simulink model "TangapCumTaoTai_2023b"  (R2023b)
settings: Solver=FixedStepAuto  StartTime=0  StopTime=350.02  FixedStep=0.00025  RelTol=1e-3  AbsTol=1e-3  EnableMultiTasking=on
undefined symbols (not defined in the file): Lg, rad, Rg, s
libraries: aerolibconvert2 x1, SignalEditorBlockLib x1
settings Model: Creator=Admin  LastModifiedBy=Legion
settings SolverCC: AutoScaleAbsTol=off  AlgebraicLoopSolver=TrustRegion  MaxZcPerStep=1
settings DataIOCC: LimitDataPoints=on  MaxDataPoints=10000
settings OptimizationCC: ReuseModelBlockBuffer=off  LifeSpan=inf
settings DebuggingCC: UnconnectedInputMsg=warning  UnconnectedOutputMsg=warning  UnconnectedLineMsg=warning  AllowSymbolicDim=off  SubsystemReferenceDiagnosticForUnitTest=warning  SFUnexpectedBacktrackingDiag=warning  SFNoUnconditionalDefaultTransitionDiag=warning  SFExecutionAtInitializationDiag=none  ArithmeticOperatorsInVariantConditions=warning
settings ModelReferenceCC: EnableRefExpFcnMdlSchedulingChecks=on
settings SFSimCC: SimUseLocalCustomCode=off  CustomCodeUndefinedFunction=UseInterfaceOnly
settings RTWCC: RTWUseLocalCustomCode=off  DLArmComputeVersion=19.05
settings CodeAppCC: StateflowObjectComments=on
settings GRTTargetCC: TargetLangStandard=C89/C90 (ANSI)
settings ConfigComp: CovMetricSettings=dw  CovSaveCumulativeToWorkspaceVar=on  CovSaveSingleToWorkspaceVar=on  CovExternalEMLEnable=off  CovSFcnEnable=off
settings SimscapeCC: SimscapeLogType=all  SimscapeLogSimulationStatistics=on  SimscapeLogDataHistory=10000

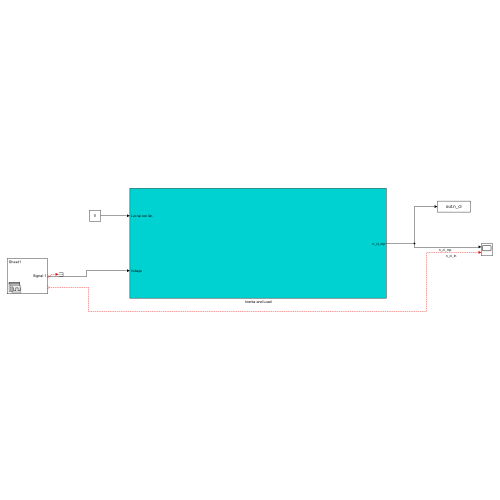
[thumbnail: Simulink's stored preview of the top-level diagram]
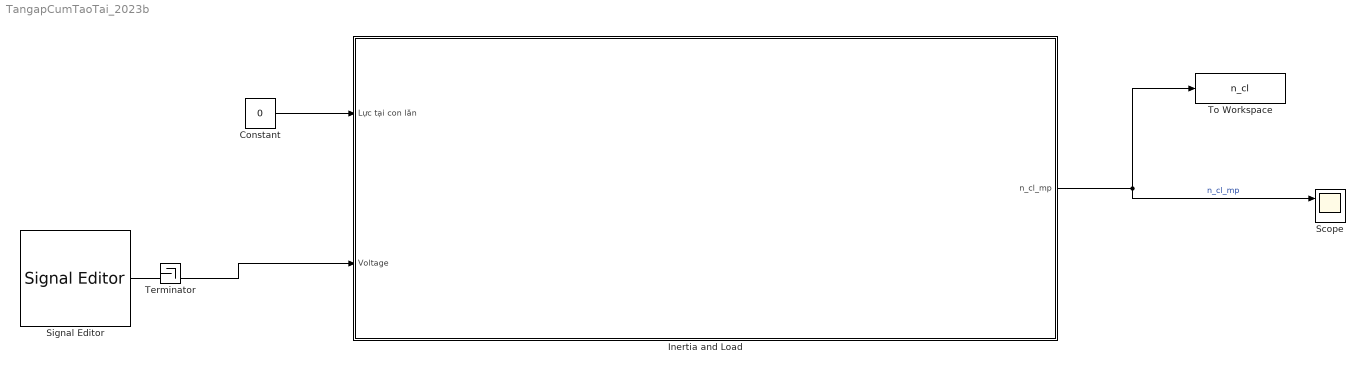
== system TangapCumTaoTai_2023b ==
  " Inertia and Load" : Subsystem
  Constant : Constant  Value=0
  Scope : Scope  NumInputPorts=2
  Signal Editor : SignalEditorBlockLib/Signal Editor  FileName=DataTangapcumtaotai.mat  ActiveScenario=Sheet1  ActiveSignal=Voltage  IsBus=off  OutputBusObjectStr=Bus: BusObject  SampleTime=0  ZeroCross=off  OutputAfterFinalValue=Setting to zero  Unit=inherit  PreserveSignalName=on  ApplySigPropsToAllScenarios=on  ApplySigPropsToAllSignals=off
  Terminator : Terminator
  To Workspace : ToWorkspace  VariableName=n_cl  SaveFormat=Timeseries  SampleTime=-1
  wires:
  Constant/1 -> " Inertia and Load"/1(Lực tại con lăn)
  Signal Editor/1 -> " Inertia and Load"/2(Voltage)
  ? -> Terminator/1
  " Inertia and Load"/1(n_cl_mp) -> To Workspace/1, Scope/1  "n_cl_mp"
  ? -> Scope/2  "n_cl_tn"

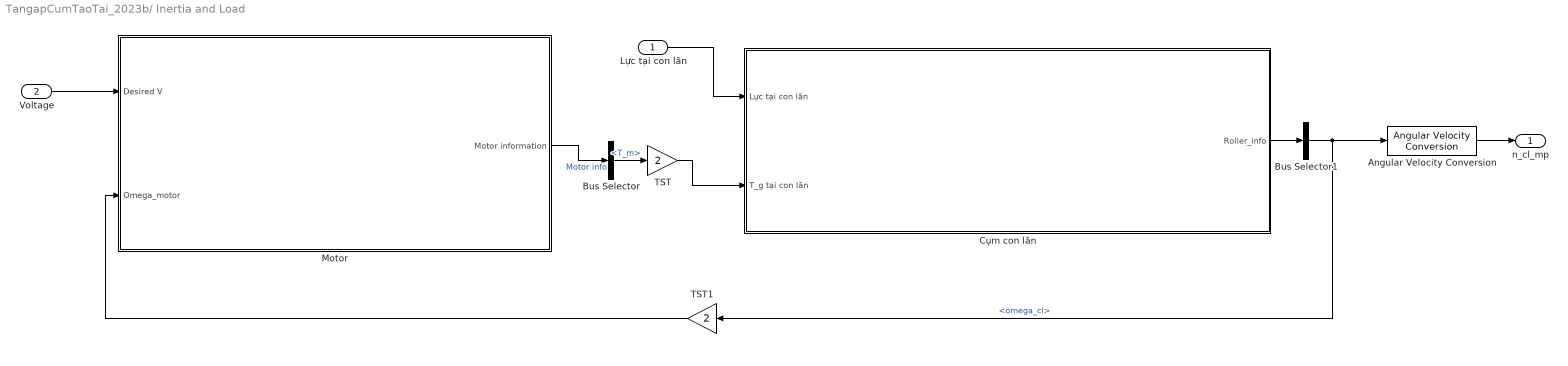
== system TangapCumTaoTai_2023b/ Inertia and Load ==
  Lực tại con lăn : Inport
  Voltage : Inport  Port=2
  Angular Velocity Conversion : aerolibconvert2/Angular Velocity Conversion  IU=rad/s  OU=rpm
  Bus Selector : BusSelector  OutputSignals=T_m
  Bus Selector1 : BusSelector  OutputSignals=omega_cl
  Cụm con lăn : Subsystem
  Motor : Subsystem
  TST : Gain  Gain=2
  TST1 : Gain  Gain=2
  n_cl_mp : Outport
  wires:
  Lực tại con lăn/1 -> Cụm con lăn/1(Lực tại con lăn)
  TST/1 -> Cụm con lăn/2(T_g tại con lăn)
  Motor/1(Motor information) -> Bus Selector/1  "Motor info"
  Bus Selector/1 -> TST/1  "<T_m>"
  Voltage/1 -> Motor/1(" Desired V")
  Cụm con lăn/1(Roller_info) -> Bus Selector1/1
  Bus Selector1/1 -> Angular Velocity Conversion/1, TST1/1  "<omega_cl>"
  TST1/1 -> Motor/2(Omega_motor)
  Angular Velocity Conversion/1 -> n_cl_mp/1

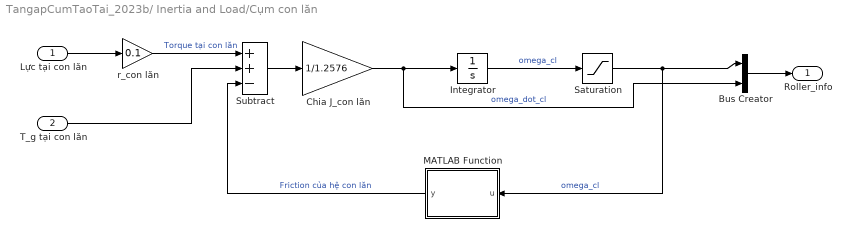
== system TangapCumTaoTai_2023b/ Inertia and Load/Cụm con lăn ==
  Lực tại con lăn : Inport
  T_g tại con lăn : Inport  Port=2
  Bus Creator : BusCreator  Inputs=2
  Chia J_con lăn : Gain  Gain=1/1.2576
  Integrator : Integrator  LimitOutput=on  LowerSaturationLimit=0
  MATLAB Function : MATLAB Function  TreatAsAtomicUnit=on
  Saturation : Saturate  UpperLimit=inf  LowerLimit=0
  Subtract : Sum  Inputs=++-
  r_con lăn : Gain  Gain=0.1
  Roller_info : Outport
  wires:
  Subtract/1 -> Chia J_con lăn/1
  r_con lăn/1 -> Subtract/1  "Torque tại con lăn"
  Saturation/1 -> Bus Creator/1, MATLAB Function/1(u)  "omega_cl"
  Integrator/1 -> Saturation/1  "omega_cl"
  Chia J_con lăn/1 -> Bus Creator/2, Integrator/1  "omega_dot_cl"
  MATLAB Function/1(y) -> Subtract/3  "Friction của hệ con lăn"
  T_g tại con lăn/1 -> Subtract/2
  Lực tại con lăn/1 -> r_con lăn/1
  Bus Creator/1 -> Roller_info/1

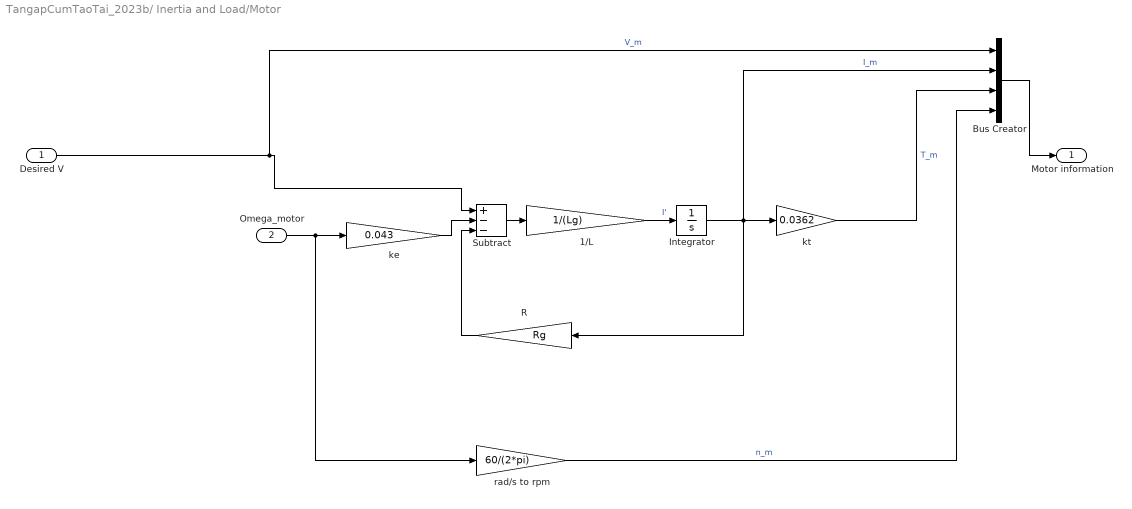
== system TangapCumTaoTai_2023b/ Inertia and Load/Motor ==
  " Desired V" : Inport
  Omega_motor : Inport  Port=2
  1/L : Gain  Gain=1/(Lg)
  Bus Creator : BusCreator  Inputs=4
  Integrator : Integrator
  R : Gain  Gain=Rg
  Subtract : Sum  Inputs=+--
  ke : Gain  Gain=0.043
  kt : Gain  Gain=0.0362
  rad/s to rpm : Gain  Gain=60/(2*pi)
  Motor information : Outport
  wires:
  Omega_motor/1 -> rad/s to rpm/1, ke/1
  R/1 -> Subtract/3
  ke/1 -> Subtract/2
  Subtract/1 -> 1/L/1
  1/L/1 -> Integrator/1  "I'"
  Integrator/1 -> Bus Creator/2, R/1, kt/1  "I_m"
  Bus Creator/1 -> Motor information/1
  " Desired V"/1 -> Subtract/1, Bus Creator/1  "V_m"
  kt/1 -> Bus Creator/3  "T_m"
  rad/s to rpm/1 -> Bus Creator/4  "n_m"

== matlab function TangapCumTaoTai_2023b/ Inertia and Load/Cụm con lăn/MATLAB Function ==
  data: u input; y output
function y = fcn(u)

y = 0.0362*(0.0601*u+8.2494)*2;
